simulink model "TST_HPUn_Co"  (R2016b)
settings: Solver=FixedStepDiscrete  StartTime=0.0  StopTime=simTime  FixedStep=sampleTime  RelTol=1e-3
values from neighbouring files (symbols this model uses):
  testCase = 1    [initTST_HPUn_Co_001.m]
libraries: simulink x6, UnitTest_Lib x4
settings Model: Creator=zhengjinyan  LastModifiedBy=zhengjinyan
settings DebuggingCC: SignalRangeChecking=error

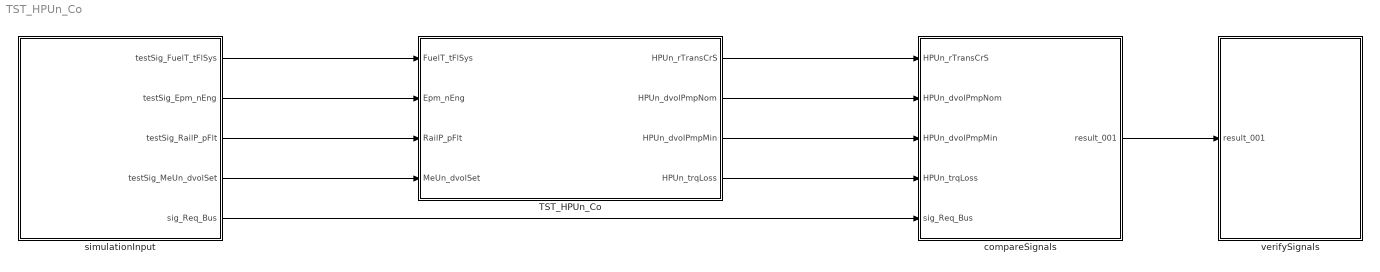
== system TST_HPUn_Co ==
  TST_HPUn_Co : Subsystem
  compareSignals : Subsystem
  simulationInput : Subsystem
  verifySignals : Subsystem
  wires:
  simulationInput/1(testSig_FuelT_tFlSys) -> TST_HPUn_Co/1(FuelT_tFlSys)
  simulationInput/2(testSig_Epm_nEng) -> TST_HPUn_Co/2(Epm_nEng)
  simulationInput/3(testSig_RailP_pFlt) -> TST_HPUn_Co/3(RailP_pFlt)
  simulationInput/4(testSig_MeUn_dvolSet) -> TST_HPUn_Co/4(MeUn_dvolSet)
  TST_HPUn_Co/1(HPUn_rTransCrS) -> compareSignals/1(HPUn_rTransCrS)
  TST_HPUn_Co/2(HPUn_dvolPmpNom) -> compareSignals/2(HPUn_dvolPmpNom)
  TST_HPUn_Co/3(HPUn_dvolPmpMin) -> compareSignals/3(HPUn_dvolPmpMin)
  TST_HPUn_Co/4(HPUn_trqLoss) -> compareSignals/4(HPUn_trqLoss)
  simulationInput/5(sig_Req_Bus) -> compareSignals/5(sig_Req_Bus)
  compareSignals/1(result_001) -> verifySignals/1(result_001)

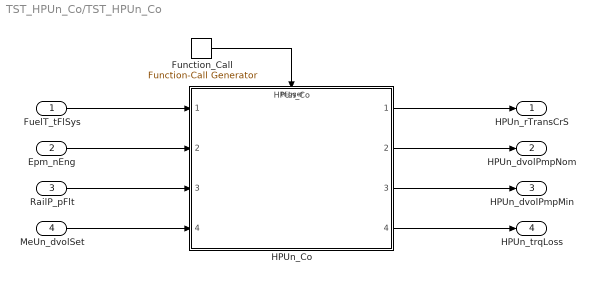
== system TST_HPUn_Co/TST_HPUn_Co ==
  FuelT_tFlSys : Inport
  Epm_nEng : Inport  Port=2
  RailP_pFlt : Inport  Port=3
  MeUn_dvolSet : Inport  Port=4
  Function_Call : simulink/Ports & Subsystems/Function-Call Generator  sample_time=sampleTime  numberOfIterations=1
  HPUn_Co : ModelReference  ModelNameDialog=HPUn_Co  SimulationMode=Normal  ModelReferenceVersion=1.28  TriggerPortName=function  TriggerPortTriggerType=function-call  TriggerPortStatesWhenEnabling=held
  HPUn_rTransCrS : Outport
  HPUn_dvolPmpNom : Outport  Port=2
  HPUn_dvolPmpMin : Outport  Port=3
  HPUn_trqLoss : Outport  Port=4
  wires:
  Function_Call/1 -> HPUn_Co/Trigger
  FuelT_tFlSys/1 -> HPUn_Co/1
  Epm_nEng/1 -> HPUn_Co/2
  RailP_pFlt/1 -> HPUn_Co/3
  MeUn_dvolSet/1 -> HPUn_Co/4
  HPUn_Co/1 -> HPUn_rTransCrS/1
  HPUn_Co/2 -> HPUn_dvolPmpNom/1
  HPUn_Co/3 -> HPUn_dvolPmpMin/1
  HPUn_Co/4 -> HPUn_trqLoss/1

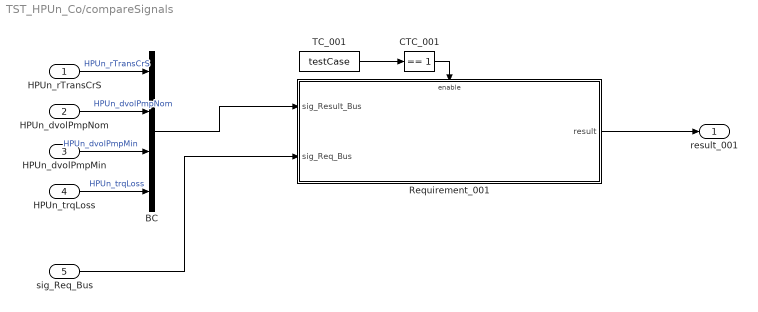
== system TST_HPUn_Co/compareSignals ==
  HPUn_rTransCrS : Inport
  HPUn_dvolPmpNom : Inport  Port=2
  HPUn_dvolPmpMin : Inport  Port=3
  HPUn_trqLoss : Inport  Port=4
  sig_Req_Bus : Inport  Port=5
  BC : BusCreator  Inputs=4
  CTC_001 : simulink/Logic and Bit Operations/Compare To Constant  relop===  const=1  OutDataTypeStr=boolean
  Requirement_001 : Subsystem
  TC_001 : Constant  Value=testCase
  result_001 : Outport
  wires:
  HPUn_rTransCrS/1 -> BC/1  "HPUn_rTransCrS"
  HPUn_dvolPmpNom/1 -> BC/2  "HPUn_dvolPmpNom"
  HPUn_dvolPmpMin/1 -> BC/3  "HPUn_dvolPmpMin"
  HPUn_trqLoss/1 -> BC/4  "HPUn_trqLoss"
  TC_001/1 -> CTC_001/1
  CTC_001/1 -> Requirement_001/Enable
  sig_Req_Bus/1 -> Requirement_001/2(sig_Req_Bus)
  BC/1 -> Requirement_001/1(sig_Result_Bus)
  Requirement_001/1(result) -> result_001/1

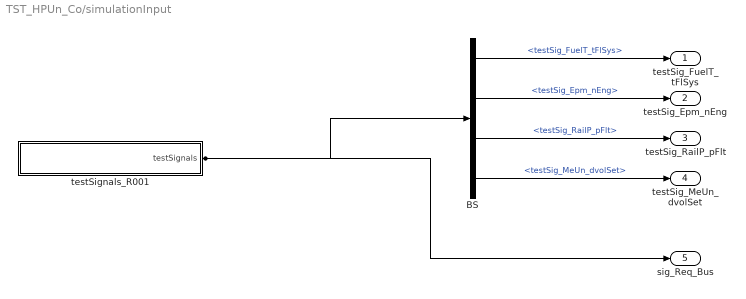
== system TST_HPUn_Co/simulationInput ==
  BS : BusSelector  OutputSignals=testSig_FuelT_tFlSys,testSig_Epm_nEng,testSig_RailP_pFlt,testSig_MeUn_dvolSet
  testSignals_R001 : Subsystem
  testSig_FuelT_tFlSys : Outport
  testSig_Epm_nEng : Outport  Port=2
  testSig_RailP_pFlt : Outport  Port=3
  testSig_MeUn_dvolSet : Outport  Port=4
  sig_Req_Bus : Outport  Port=5
  wires:
  BS/1 -> testSig_FuelT_tFlSys/1  "<testSig_FuelT_tFlSys>"
  BS/2 -> testSig_Epm_nEng/1  "<testSig_Epm_nEng>"
  BS/3 -> testSig_RailP_pFlt/1  "<testSig_RailP_pFlt>"
  BS/4 -> testSig_MeUn_dvolSet/1  "<testSig_MeUn_dvolSet>"
  testSignals_R001/1(testSignals) -> BS/1, sig_Req_Bus/1

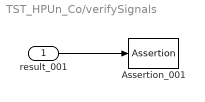
== system TST_HPUn_Co/verifySignals ==
  result_001 : Inport
  Assertion_001 : Assertion  Enabled=off
  wires:
  result_001/1 -> Assertion_001/1

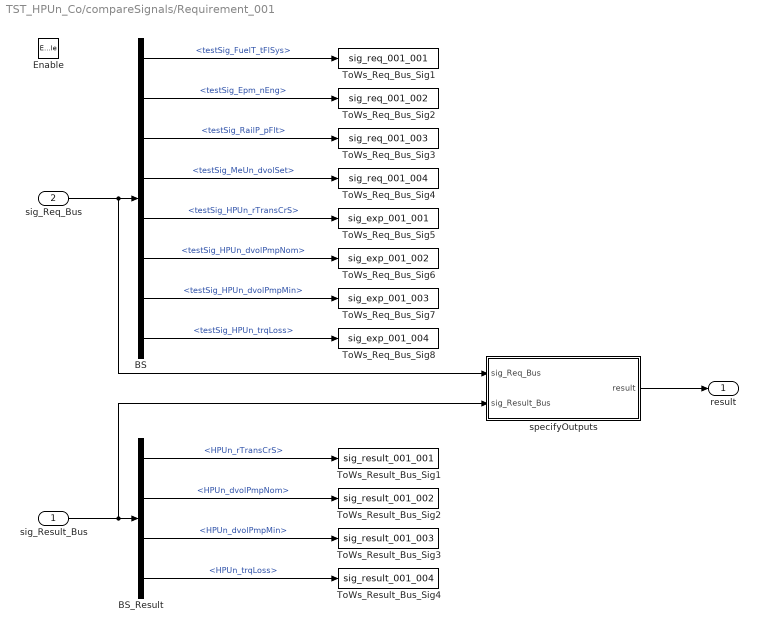
== system TST_HPUn_Co/compareSignals/Requirement_001 ==
  sig_Result_Bus : Inport
  sig_Req_Bus : Inport  Port=2
  Enable : EnablePort
  BS : BusSelector  OutputSignals=testSig_FuelT_tFlSys,testSig_Epm_nEng,testSig_RailP_pFlt,testSig_MeUn_dvolSet,testSig_HPUn_rTransCrS,testSig_HPUn_dvolPmpNom,testSig_HPUn_dvolPmpMin,testSig_HPUn_trqLoss
  BS_Result : BusSelector  OutputSignals=HPUn_rTransCrS,HPUn_dvolPmpNom,HPUn_dvolPmpMin,HPUn_trqLoss
  ToWs_Req_Bus_Sig1 : ToWorkspace  VariableName=sig_req_001_001  SaveFormat=Structure With Time
  ToWs_Req_Bus_Sig2 : ToWorkspace  VariableName=sig_req_001_002  SaveFormat=Structure With Time
  ToWs_Req_Bus_Sig3 : ToWorkspace  VariableName=sig_req_001_003  SaveFormat=Structure With Time
  ToWs_Req_Bus_Sig4 : ToWorkspace  VariableName=sig_req_001_004  SaveFormat=Structure With Time
  ToWs_Req_Bus_Sig5 : ToWorkspace  VariableName=sig_exp_001_001  SaveFormat=Structure With Time
  ToWs_Req_Bus_Sig6 : ToWorkspace  VariableName=sig_exp_001_002  SaveFormat=Structure With Time
  ToWs_Req_Bus_Sig7 : ToWorkspace  VariableName=sig_exp_001_003  SaveFormat=Structure With Time
  ToWs_Req_Bus_Sig8 : ToWorkspace  VariableName=sig_exp_001_004  SaveFormat=Structure With Time
  ToWs_Result_Bus_Sig1 : ToWorkspace  VariableName=sig_result_001_001  SaveFormat=Structure With Time
  ToWs_Result_Bus_Sig2 : ToWorkspace  VariableName=sig_result_001_002  SaveFormat=Structure With Time
  ToWs_Result_Bus_Sig3 : ToWorkspace  VariableName=sig_result_001_003  SaveFormat=Structure With Time
  ToWs_Result_Bus_Sig4 : ToWorkspace  VariableName=sig_result_001_004  SaveFormat=Structure With Time
  specifyOutputs : Subsystem
  result : Outport
  wires:
  sig_Req_Bus/1 -> BS/1, specifyOutputs/1(sig_Req_Bus)
  BS/1 -> ToWs_Req_Bus_Sig1/1  "<testSig_FuelT_tFlSys>"
  BS/2 -> ToWs_Req_Bus_Sig2/1  "<testSig_Epm_nEng>"
  BS/3 -> ToWs_Req_Bus_Sig3/1  "<testSig_RailP_pFlt>"
  BS/4 -> ToWs_Req_Bus_Sig4/1  "<testSig_MeUn_dvolSet>"
  BS/5 -> ToWs_Req_Bus_Sig5/1  "<testSig_HPUn_rTransCrS>"
  BS/6 -> ToWs_Req_Bus_Sig6/1  "<testSig_HPUn_dvolPmpNom>"
  BS/7 -> ToWs_Req_Bus_Sig7/1  "<testSig_HPUn_dvolPmpMin>"
  BS/8 -> ToWs_Req_Bus_Sig8/1  "<testSig_HPUn_trqLoss>"
  sig_Result_Bus/1 -> BS_Result/1, specifyOutputs/2(sig_Result_Bus)
  BS_Result/1 -> ToWs_Result_Bus_Sig1/1  "<HPUn_rTransCrS>"
  BS_Result/2 -> ToWs_Result_Bus_Sig2/1  "<HPUn_dvolPmpNom>"
  BS_Result/3 -> ToWs_Result_Bus_Sig3/1  "<HPUn_dvolPmpMin>"
  BS_Result/4 -> ToWs_Result_Bus_Sig4/1  "<HPUn_trqLoss>"
  specifyOutputs/1(result) -> result/1

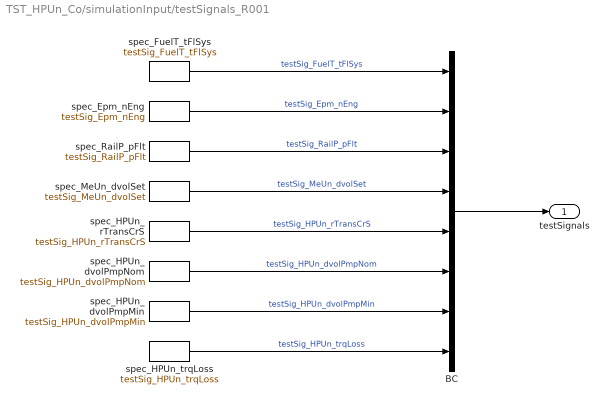
== system TST_HPUn_Co/simulationInput/testSignals_R001 ==
  BC : BusCreator  Inputs=8
  spec_Epm_nEng : FromWorkspace  VariableName=testSig_Epm_nEng  Interpolate=off  OutputAfterFinalValue=Holding final value
  spec_FuelT_tFlSys : FromWorkspace  VariableName=testSig_FuelT_tFlSys  Interpolate=off  OutputAfterFinalValue=Holding final value
  spec_HPUn_dvolPmpMin : FromWorkspace  VariableName=testSig_HPUn_dvolPmpMin  Interpolate=off  OutputAfterFinalValue=Holding final value
  spec_HPUn_dvolPmpNom : FromWorkspace  VariableName=testSig_HPUn_dvolPmpNom  Interpolate=off  OutputAfterFinalValue=Holding final value
  spec_HPUn_rTransCrS : FromWorkspace  VariableName=testSig_HPUn_rTransCrS  Interpolate=off  OutputAfterFinalValue=Holding final value
  spec_HPUn_trqLoss : FromWorkspace  VariableName=testSig_HPUn_trqLoss  Interpolate=off  OutputAfterFinalValue=Holding final value
  spec_MeUn_dvolSet : FromWorkspace  VariableName=testSig_MeUn_dvolSet  Interpolate=off  OutputAfterFinalValue=Holding final value
  spec_RailP_pFlt : FromWorkspace  VariableName=testSig_RailP_pFlt  Interpolate=off  OutputAfterFinalValue=Holding final value
  testSignals : Outport
  wires:
  BC/1 -> testSignals/1
  spec_FuelT_tFlSys/1 -> BC/1  "testSig_FuelT_tFlSys"
  spec_Epm_nEng/1 -> BC/2  "testSig_Epm_nEng"
  spec_RailP_pFlt/1 -> BC/3  "testSig_RailP_pFlt"
  spec_MeUn_dvolSet/1 -> BC/4  "testSig_MeUn_dvolSet"
  spec_HPUn_rTransCrS/1 -> BC/5  "testSig_HPUn_rTransCrS"
  spec_HPUn_dvolPmpNom/1 -> BC/6  "testSig_HPUn_dvolPmpNom"
  spec_HPUn_dvolPmpMin/1 -> BC/7  "testSig_HPUn_dvolPmpMin"
  spec_HPUn_trqLoss/1 -> BC/8  "testSig_HPUn_trqLoss"

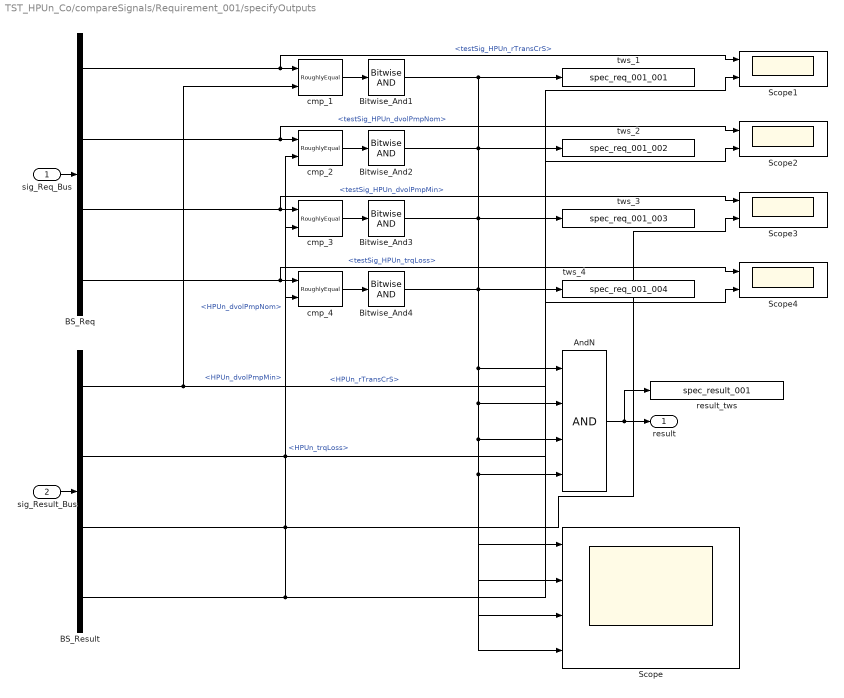
== system TST_HPUn_Co/compareSignals/Requirement_001/specifyOutputs ==
  sig_Req_Bus : Inport
  sig_Result_Bus : Inport  Port=2
  AndN : Logic  Inputs=4
  BS_Req : BusSelector  OutputSignals=testSig_HPUn_rTransCrS,testSig_HPUn_dvolPmpNom,testSig_HPUn_dvolPmpMin,testSig_HPUn_trqLoss
  BS_Result : BusSelector  OutputSignals=HPUn_rTransCrS,HPUn_dvolPmpNom,HPUn_dvolPmpMin,HPUn_trqLoss
  Bitwise_And{1..4} (4 alike) : simulink/Logic and Bit Operations/Bitwise Operator  logicop=AND  UseBitMask=off  BitMask=bin2dec('11011001')  BitMaskRealWorld=Stored Integer
  Scope : Scope  NumInputPorts=4
  Scope{1..4} (4 alike) : Scope  NumInputPorts=2
  cmp_1 : UnitTest_Lib/RoughlyEqual  slope=0.1
  cmp_2 : UnitTest_Lib/RoughlyEqual  slope=20
  cmp_3 : UnitTest_Lib/RoughlyEqual  slope=20
  cmp_4 : UnitTest_Lib/RoughlyEqual  slope=0.1
  result_tws : ToWorkspace  VariableName=spec_result_001
  tws_1 : ToWorkspace  VariableName=spec_req_001_001
  tws_2 : ToWorkspace  VariableName=spec_req_001_002
  tws_3 : ToWorkspace  VariableName=spec_req_001_003
  tws_4 : ToWorkspace  VariableName=spec_req_001_004
  result : Outport
  wires:
  sig_Req_Bus/1 -> BS_Req/1
  sig_Result_Bus/1 -> BS_Result/1
  AndN/1 -> result/1, result_tws/1
  BS_Req/1 -> cmp_1/1, Scope1/1  "<testSig_HPUn_rTransCrS>"
  BS_Result/1 -> cmp_1/2, Scope1/2  "<HPUn_rTransCrS>"
  cmp_1/1 -> Bitwise_And1/1
  Bitwise_And1/1 -> AndN/1, Scope/1, tws_1/1
  BS_Req/2 -> cmp_2/1, Scope2/1  "<testSig_HPUn_dvolPmpNom>"
  BS_Result/2 -> cmp_2/2, Scope2/2  "<HPUn_dvolPmpNom>"
  cmp_2/1 -> Bitwise_And2/1
  Bitwise_And2/1 -> AndN/2, Scope/2, tws_2/1
  BS_Req/3 -> cmp_3/1, Scope3/1  "<testSig_HPUn_dvolPmpMin>"
  BS_Result/3 -> cmp_3/2, Scope3/2  "<HPUn_dvolPmpMin>"
  cmp_3/1 -> Bitwise_And3/1
  Bitwise_And3/1 -> AndN/3, Scope/3, tws_3/1
  BS_Req/4 -> cmp_4/1, Scope4/1  "<testSig_HPUn_trqLoss>"
  BS_Result/4 -> cmp_4/2, Scope4/2  "<HPUn_trqLoss>"
  cmp_4/1 -> Bitwise_And4/1
  Bitwise_And4/1 -> AndN/4, Scope/4, tws_4/1
